simulink model "simulink_FCS_SDA"  (R2023a)
settings: Solver=VariableStepAuto  StartTime=0.0  StopTime=3*(1/freqHzSin)  FixedStep=Ts  RelTol=1e-3
InitFcn:
  | v0_setupFCS
StopFcn:
  | % t = table(out.seq, out.t_sim, 'VariableNames', ["Sequência de Vetores","Tempo de Simulação"]);
  | % writetable(t,'C:\Users\jpbru\OneDrive\Documentos\UFSC\COBEP 2023\sequencia_states.xlsx','Sheet','sim_CF_gw')
  | % winopen('C:\Users\jpbru\OneDrive\Documentos\UFSC\COBEP 2023\sequencia_states.xlsx')
  | %
  | % nome_arq = sprintf("gdq_caso-1_7.csv");
  | % writematrix([out.y_d out.y_q out.y_a out.y_b out.y_c out.ref_a out.ref_b out.ref_c],"C:\Users\jpbru\OneDrive\Documentos\MATLAB\CPBM\TrabFinal\Etapa 9 - Setembro2023 -\graficos\"+nome_arq)
  | 
  | sprintf("MSE = %.3f", out.mse)
  | sprintf("THD = %.3f", out.thd)
  | sprintf("Niter_avg = %d", round(out.Niter_avg))
  | % sprintf("Csw = %.0f", out.csw)
  | % sprintf("Tempo de Computo = %.3fms", out.tavg*1000)
values from neighbouring files (symbols this model uses):
  A = [A1; A2]    [v0_setupFCS.m]
  B = [B1; B2; B3; B4; B5; B6]    [v0_setupFCS.m]
  Csim = C*(1-P/100)    (= 5e-05)    [v0_setupFCS.m]
  dimA = length(A1)    [v0_setupFCS.m]
  dimB = length(B1)    [v0_setupFCS.m]
  freqHzSin = 50    [v0_setupFCS.m]
  Lsim = L*(1-P/100)    (= 0.002)    [v0_setupFCS.m]
  N = 4    [v0_setupFCS.m]
  N1 = 2    [v0_setupFCS.m]
  N2 = N+N1-1    (= 5)    [v0_setupFCS.m]
  Rsim = R*(1-P/100)    (= 60)    [v0_setupFCS.m]
  Ts = 1/Fs    (= 5e-05)    [v0_setupFCS.m]
  Vdc_sim = Vdc*1    (= 400)    [v0_setupFCS.m]
  vectors = [ 0   0   0 ... (first row only)    [v0_setupFCS.m]
  Vnoise = 0    [v0_setupFCS.m]
  Vo_ref_amp = 120*sqrt(2)    [v0_setupFCS.m]
undefined symbols (not defined in the file or in its folder): DiscIntNeverNeededParam, Lfilter
libraries: dspstat3 x10, spsSeriesRLCBranchLib x9, spsVoltageMeasurementLib x7, spsCurrentMeasurementLib x6, spsIdealSwitchLib x6, spsTHDLib x4, spsabctoAlphaBetaZeroLib x4, simulink x2, spsControlledVoltageSourceLib x1, sps_lib x1
settings Model: Creator=jpbru  LastModifiedBy=jpbru
settings SolverCC: AlgebraicLoopSolver=TrustRegion
settings DebuggingCC: UnconnectedInputMsg=warning  UnconnectedOutputMsg=warning  UnconnectedLineMsg=warning
settings ModelReferenceCC: EnableRefExpFcnMdlSchedulingChecks=on

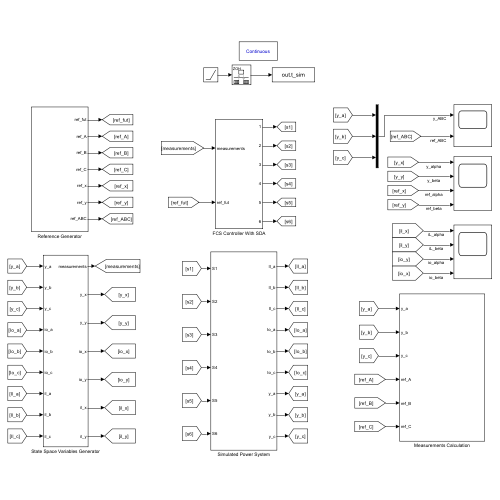
[thumbnail: Simulink's stored preview of the top-level diagram]
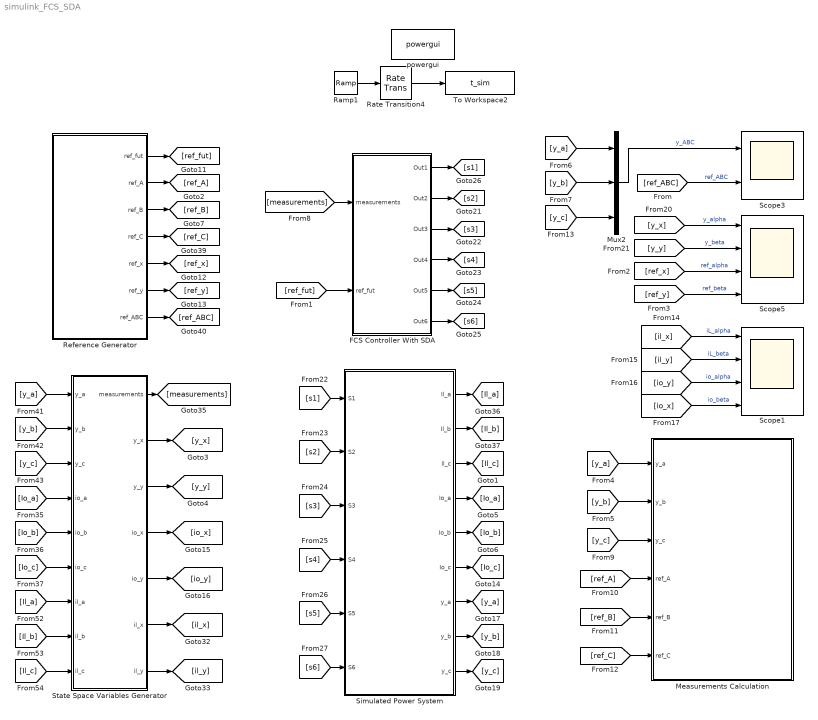
== system simulink_FCS_SDA ==
  FCS Controller With SDA : Subsystem
  Measurements Calculation : Subsystem
  Mux2 : Mux  Inputs=3
  Ramp1 : simulink/Sources/Ramp  slope=1  start=0  InitialOutput=0
  Rate Transition4 : RateTransition  OutPortSampleTime=Ts
  Reference Generator : Subsystem
  Scope1 : Scope  NumInputPorts=4
  Scope3 : Scope  NumInputPorts=2
  Scope5 : Scope  NumInputPorts=4
  Simulated Power System : Subsystem
  State Space Variables Generator : Subsystem
  To Workspace2 : ToWorkspace  VariableName=t_sim  SampleTime=Ts
      settings: Save2DSignal=2-D array (concatenate along first dimension)
  powergui : sps_lib/powergui  Priority=1  SimulationMode=Continuous  SampleTime=Ts  frequency=60  Iterations=50  frequencyindice=0  Pbase=100e6  ErrMax=1e-4  UnitsV=kV  UnitsW=MW  buscounter=0  FunctionMessages=off  echomessages=off  EnableUseOfTLC=off  CurrentSourceSwitches=off  DisableSnubberDevices=off  DisableRonSwitches=off  DisableVfSwitches=off  DisplayEquations=off  AutomaticDiscreteSolvers=off  SolverType=Tustin/Backward Euler (TBE)  Interpol=off  ExternalGateDelay=off  methode=off  Ts=100  x0status=blocks  SPID=on  SwTol=0  HookPort=off  NonlinearTolerance=1e-4  nMaxIteration=100  ContinueOnMaxIteration=off  RestoreLinks=warning  ResistiveCurrentMeasurement=off  Frange=[0:2:500]  Ylog=off  Xlog=on  ShowGrid=off  save=off  variable=ZData  structure=0  ZoomFFT=off  StartTime=0.0  cycles=1  DisplayStyle=1  fundamental=60  FreqAxis=off  MaxFrequency=1000  frequencyindicesteady=1  RmsSteady=1  display=off
  wires:
  [ref_y] -> Scope5/4  "ref_beta"
  [y_a] -> Mux2/1
  [y_b] -> Mux2/2
  [y_c] -> Mux2/3
  Mux2/1 -> Scope3/1  "y_ABC"
  [y_x] -> Scope5/1  "y_alpha"
  [y_y] -> Scope5/2  "y_beta"
  [ref_x] -> Scope5/3  "ref_alpha"
  Ramp1/1 -> Rate Transition4/1
  Rate Transition4/1 -> To Workspace2/1
  Reference Generator/1(ref_fut) -> [ref_fut]
  Reference Generator/2(ref_A) -> [ref_A]
  Reference Generator/3(ref_B) -> [ref_B]
  Reference Generator/4(ref_C) -> [ref_C]
  Reference Generator/6(ref_y) -> [ref_y]
  Reference Generator/5(ref_x) -> [ref_x]
  [y_a] -> State Space Variables Generator/1(y_a)
  [y_b] -> State Space Variables Generator/2(y_b)
  [y_c] -> State Space Variables Generator/3(y_c)
  [Io_a] -> State Space Variables Generator/4(io_a)
  [Io_b] -> State Space Variables Generator/5(io_b)
  [Io_c] -> State Space Variables Generator/6(io_c)
  [Il_a] -> State Space Variables Generator/7(il_a)
  [Il_b] -> State Space Variables Generator/8(il_b)
  [Il_c] -> State Space Variables Generator/9(il_c)
  State Space Variables Generator/1(measurements) -> [measurements]
  State Space Variables Generator/4(io_x) -> [io_x]
  State Space Variables Generator/5(io_y) -> [io_y]
  State Space Variables Generator/6(il_x) -> [il_x]
  State Space Variables Generator/7(il_y) -> [il_y]
  State Space Variables Generator/3(y_y) -> [y_y]
  State Space Variables Generator/2(y_x) -> [y_x]
  Reference Generator/7(ref_ABC) -> [ref_ABC]
  [ref_ABC] -> Scope3/2  "ref_ABC"
  [measurements] -> FCS Controller With SDA/1(measurements)
  [ref_fut] -> FCS Controller With SDA/2(ref_fut)
  FCS Controller With SDA/1(Out1) -> [s1]
  FCS Controller With SDA/2(Out2) -> [s2]
  FCS Controller With SDA/3(Out3) -> [s3]
  FCS Controller With SDA/4(Out4) -> [s4]
  FCS Controller With SDA/5(Out5) -> [s5]
  FCS Controller With SDA/6(Out6) -> [s6]
  [s1] -> Simulated Power System/1(S1)
  Simulated Power System/9(y_c) -> [y_c]
  Simulated Power System/8(y_b) -> [y_b]
  Simulated Power System/7(y_a) -> [y_a]
  [s2] -> Simulated Power System/2(S2)
  [s3] -> Simulated Power System/3(S3)
  [s4] -> Simulated Power System/4(S4)
  [s5] -> Simulated Power System/5(S5)
  [s6] -> Simulated Power System/6(S6)
  Simulated Power System/1(Il_a) -> [Il_a]
  Simulated Power System/2(Il_b) -> [Il_b]
  Simulated Power System/3(Il_c) -> [Il_c]
  Simulated Power System/4(Io_a) -> [Io_a]
  Simulated Power System/5(Io_b) -> [Io_b]
  Simulated Power System/6(Io_c) -> [Io_c]
  [ref_C] -> Measurements Calculation/6(ref_C)
  [ref_B] -> Measurements Calculation/5(ref_B)
  [ref_A] -> Measurements Calculation/4(ref_A)
  [y_c] -> Measurements Calculation/3(y_c)
  [y_b] -> Measurements Calculation/2(y_b)
  [y_a] -> Measurements Calculation/1(y_a)
  [il_x] -> Scope1/1  "iL_alpha"
  [il_y] -> Scope1/2  "iL_beta"
  [io_y] -> Scope1/3  "io_alpha"
  [io_x] -> Scope1/4  "io_beta"

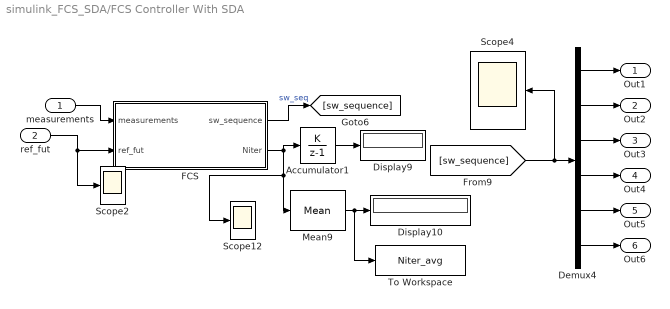
== system simulink_FCS_SDA/FCS Controller With SDA ==
  measurements : Inport
  ref_fut : Inport  Port=2
  Accumulator1 : DiscreteIntegrator  IntegratorMethod=Accumulation: Forward Euler  SampleTime=Ts  ICPrevOutput=DiscIntNeverNeededParam  ICPrevScaledInput=DiscIntNeverNeededParam
  Demux4 : Demux  Outputs=6
  Display10 : Display
  Display9 : Display
  FCS : MATLAB Function  TreatAsAtomicUnit=on  SystemSampleTime=Ts
  Mean9 : dspstat3/Mean  run=on  reset_popup=None  directionMode=Each column  dimension=1  roiEnable=off  roiType=Rectangles  roiPortion=Entire ROI  roiOutput=Individual statistics for each ROI  roiFlag=off  roundingMode=Floor  overflowMode=off  outputDataTypeStr=Inherit: Same as accumulator  outputMin=[]  outputMax=[]  outputLastDataTypeStr=Inherit: Same as accumulator
  Scope12 : Scope
  Scope2 : Scope
  Scope4 : Scope
  To Workspace : ToWorkspace  VariableName=Niter_avg  SampleTime=-1
      settings: MaxDataPoints=1
  Out1 : Outport
  Out2 : Outport  Port=2
  Out3 : Outport  Port=3
  Out4 : Outport  Port=4
  Out5 : Outport  Port=5
  Out6 : Outport  Port=6
  wires:
  Demux4/5 -> Out5/1
  [sw_sequence] -> Scope4/1, Demux4/1
  FCS/1(sw_sequence) -> [sw_sequence]  "sw_seq"
  Demux4/1 -> Out1/1
  FCS/2(Niter) -> Accumulator1/1, Scope12/1, Mean9/1
  ref_fut/1 -> Scope2/1, FCS/2(ref_fut)
  Mean9/1 -> To Workspace/1, Display10/1
  Accumulator1/1 -> Display9/1
  measurements/1 -> FCS/1(measurements)
  Demux4/3 -> Out3/1
  Demux4/2 -> Out2/1
  Demux4/6 -> Out6/1
  Demux4/4 -> Out4/1

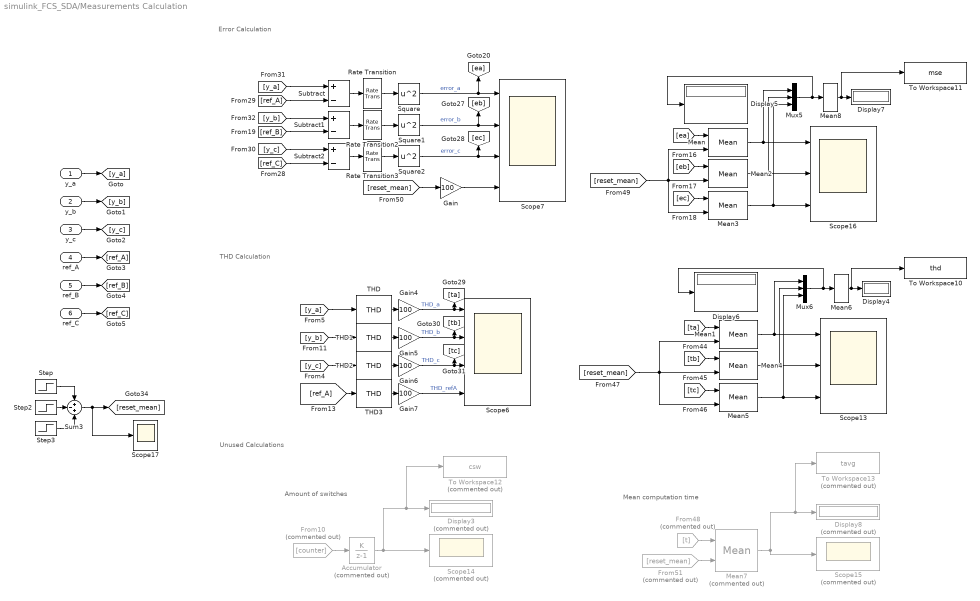
== system simulink_FCS_SDA/Measurements Calculation ==
  note: Unused Calculations
  note: THD Calculation
  note: Error Calculation
  note: Mean computation time
  note: Amount of switches
  y_a : Inport
  y_b : Inport  Port=2
  y_c : Inport  Port=3
  ref_A : Inport  Port=4
  ref_B : Inport  Port=5
  ref_C : Inport  Port=6
  Accumulator : DiscreteIntegrator  Commented=on  IntegratorMethod=Accumulation: Forward Euler  SampleTime=-1  ICPrevOutput=DiscIntNeverNeededParam  ICPrevScaledInput=DiscIntNeverNeededParam
  Display3 : Display  Commented=on
  Display{4..7} (4 alike) : Display
  Display8 : Display  Commented=on
      settings: Format=short_e
  From10 : From  Commented=on  GotoTag=counter
  From48 : From  Commented=on  GotoTag=t
  From51 : From  Commented=on  GotoTag=reset_mean
  Gain{,4..7} (5 alike) : Gain  Gain=100
  Mean{,1..5} (6 alike) : dspstat3/Mean  run=on  reset_popup=Rising edge  directionMode=Each column  dimension=1  roiEnable=off  roiType=Rectangles  roiPortion=Entire ROI  roiOutput=Individual statistics for each ROI  roiFlag=off  roundingMode=Floor  overflowMode=off  outputDataTypeStr=Inherit: Same as accumulator  outputMin=[]  outputMax=[]  outputLastDataTypeStr=Inherit: Same as accumulator
  Mean6 : dspstat3/Mean  run=off  reset_popup=Rising edge  directionMode=Entire input  dimension=1  roiEnable=off  roiType=Rectangles  roiPortion=Entire ROI  roiOutput=Individual statistics for each ROI  roiFlag=off  roundingMode=Floor  overflowMode=off  outputDataTypeStr=Inherit: Same as accumulator  outputMin=[]  outputMax=[]  outputLastDataTypeStr=Inherit: Same as accumulator
  Mean7 : dspstat3/Mean  Commented=on  run=on  reset_popup=Rising edge  directionMode=Each column  dimension=1  roiEnable=off  roiType=Rectangles  roiPortion=Entire ROI  roiOutput=Individual statistics for each ROI  roiFlag=off  roundingMode=Floor  overflowMode=off  outputDataTypeStr=Inherit: Same as accumulator  outputMin=[]  outputMax=[]  outputLastDataTypeStr=Inherit: Same as accumulator
  Mean8 : dspstat3/Mean  run=off  reset_popup=Rising edge  directionMode=Entire input  dimension=1  roiEnable=off  roiType=Rectangles  roiPortion=Entire ROI  roiOutput=Individual statistics for each ROI  roiFlag=off  roundingMode=Floor  overflowMode=off  outputDataTypeStr=Inherit: Same as accumulator  outputMin=[]  outputMax=[]  outputLastDataTypeStr=Inherit: Same as accumulator
  Mux5 : Mux  Inputs=3
  Mux6 : Mux  Inputs=3
  Rate Transition : RateTransition  OutPortSampleTime=Ts
  Rate Transition2 : RateTransition  OutPortSampleTime=Ts
  Rate Transition3 : RateTransition  OutPortSampleTime=Ts
  Scope13 : Scope  NumInputPorts=3
  Scope14 : Scope  Commented=on
  Scope15 : Scope  Commented=on
  Scope16 : Scope  NumInputPorts=3
  Scope17 : Scope
  Scope6 : Scope  NumInputPorts=4
  Scope7 : Scope  NumInputPorts=4
  Square : Math  Operator=square
  Square1 : Math  Operator=square
  Square2 : Math  Operator=square
  Step : Step  Time=(1/freqHzSin)  SampleTime=Ts
  Step2 : Step  Time=(1/freqHzSin)+Ts  SampleTime=Ts
  Step3 : Step  Time=(1/freqHzSin)*2  SampleTime=Ts
  Subtract : Sum  Inputs=+-
  Subtract1 : Sum  Inputs=+-
  Subtract2 : Sum  Inputs=+-
  Sum3 : Sum  Inputs=+-+
  THD{,1..3} (4 alike) : spsTHDLib/THD  Freq=50  Ts=Ts
  To Workspace10 : ToWorkspace  VariableName=thd  SampleTime=-1
      settings: MaxDataPoints=1
  To Workspace11 : ToWorkspace  VariableName=mse  SampleTime=-1
      settings: MaxDataPoints=1
  To Workspace12 : ToWorkspace  Commented=on  VariableName=csw  SampleTime=-1
      settings: MaxDataPoints=1
  To Workspace13 : ToWorkspace  Commented=on  VariableName=tavg  SampleTime=-1
      settings: MaxDataPoints=1
  wires:
  Rate Transition2/1 -> Square1/1
  Gain5/1 -> [tb], Scope6/2  "THD_b"
  Mean8/1 -> To Workspace11/1, Display7/1
  Mean7/1 -> To Workspace13/1, Display8/1, Scope15/1
  Subtract2/1 -> Rate Transition3/1
  Sum3/1 -> Scope17/1, [reset_mean]
  Mean6/1 -> To Workspace10/1, Display4/1
  Gain6/1 -> [tc], Scope6/3  "THD_c"
  THD2/1 -> Gain6/1
  Mux5/1 -> Mean8/1, Display5/1
  Mean3/1 -> Mux5/3, Scope16/3
  Accumulator/1 -> To Workspace12/1, Display3/1, Scope14/1
  [tc] -> Mean5/1
  [eb] -> Mean2/1
  Mux6/1 -> Display6/1, Mean6/1
  Mean5/1 -> Mux6/3, Scope13/3
  Square2/1 -> [ec], Scope7/3  "error_c"
  [ta] -> Mean1/1
  Gain4/1 -> [ta], Scope6/1  "THD_a"
  Mean1/1 -> Mux6/1, Scope13/1
  [ref_A] -> THD3/1
  [ref_C] -> Subtract2/2
  From48/1 -> Mean7/1
  Square/1 -> [ea], Scope7/1  "error_a"
  Rate Transition3/1 -> Square2/1
  [y_a] -> THD/1
  Subtract/1 -> Rate Transition/1
  [tb] -> Mean4/1
  From10/1 -> Accumulator/1
  [y_b] -> Subtract1/1
  [reset_mean] -> Mean3/2, Mean2/2, Mean/2
  Step2/1 -> Sum3/2
  Step3/1 -> Sum3/3
  [reset_mean] -> Mean1/2, Mean5/2, Mean4/2
  [reset_mean] -> Gain/1
  Mean2/1 -> Mux5/2, Scope16/2
  Mean/1 -> Mux5/1, Scope16/1
  [ec] -> Mean3/1
  [ea] -> Mean/1
  [y_b] -> THD1/1
  Gain7/1 -> Scope6/4  "THD_refA"
  [y_c] -> Subtract2/1
  Square1/1 -> [eb], Scope7/2  "error_b"
  [ref_A] -> Subtract/2
  [ref_B] -> Subtract1/2
  Subtract1/1 -> Rate Transition2/1
  THD/1 -> Gain4/1
  THD1/1 -> Gain5/1
  THD3/1 -> Gain7/1
  [y_c] -> THD2/1
  Gain/1 -> Scope7/4
  Rate Transition/1 -> Square/1
  [y_a] -> Subtract/1
  Step/1 -> Sum3/1
  From51/1 -> Mean7/2
  Mean4/1 -> Mux6/2, Scope13/2
  ref_C/1 -> [ref_C]
  ref_B/1 -> [ref_B]
  ref_A/1 -> [ref_A]
  y_c/1 -> [y_c]
  y_b/1 -> [y_b]
  y_a/1 -> [y_a]

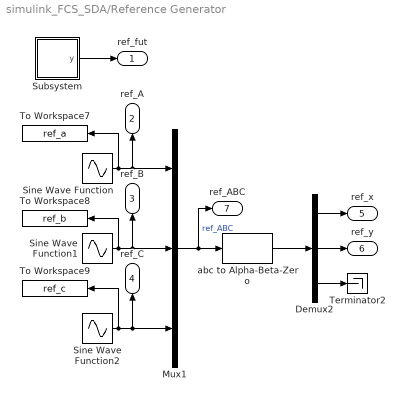
== system simulink_FCS_SDA/Reference Generator ==
  Demux2 : Demux  Outputs=3
  Mux1 : Mux  Inputs=3
  Sine Wave Function : Sin  Amplitude=Vo_ref_amp  Frequency=2*pi*50  SampleTime=Ts
  Sine Wave Function1 : Sin  Amplitude=Vo_ref_amp  Frequency=2*pi*50  Phase=-2*pi/3  SampleTime=Ts
  Sine Wave Function2 : Sin  Amplitude=Vo_ref_amp  Frequency=2*pi*50  Phase=2*pi/3  SampleTime=Ts
  Subsystem : Subsystem
  Terminator2 : Terminator
  To Workspace7 : ToWorkspace  VariableName=ref_a  SampleTime=Ts
      settings: Save2DSignal=2-D array (concatenate along first dimension)
  To Workspace8 : ToWorkspace  VariableName=ref_b  SampleTime=Ts
      settings: Save2DSignal=2-D array (concatenate along first dimension)
  To Workspace9 : ToWorkspace  VariableName=ref_c  SampleTime=Ts
      settings: Save2DSignal=2-D array (concatenate along first dimension)
  abc to Alpha-Beta-Zero : spsabctoAlphaBetaZeroLib/abc to Alpha-Beta-Zero
  ref_fut : Outport
  ref_A : Outport  Port=2
  ref_B : Outport  Port=3
  ref_C : Outport  Port=4
  ref_x : Outport  Port=5
  ref_y : Outport  Port=6
  ref_ABC : Outport  Port=7
  wires:
  Subsystem/1(y) -> ref_fut/1
  Demux2/2 -> ref_y/1
  Sine Wave Function/1 -> Mux1/1, ref_A/1, To Workspace7/1
  Demux2/3 -> Terminator2/1
  Sine Wave Function1/1 -> Mux1/2, ref_B/1, To Workspace8/1
  Demux2/1 -> ref_x/1
  Sine Wave Function2/1 -> Mux1/3, ref_C/1, To Workspace9/1
  Mux1/1 -> ref_ABC/1, abc to Alpha-Beta-Zero/1  "ref_ABC"
  abc to Alpha-Beta-Zero/1 -> Demux2/1

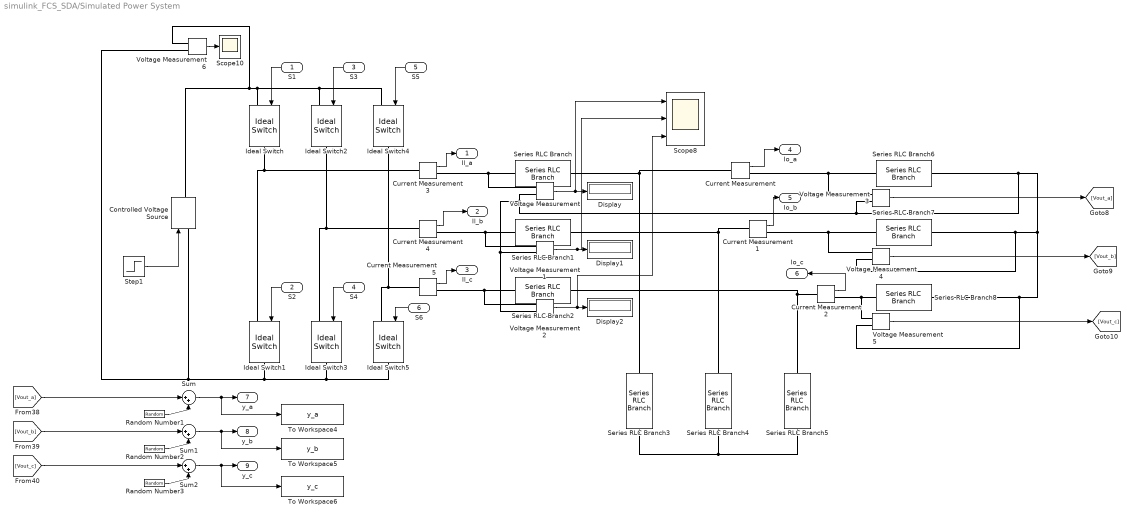
== system simulink_FCS_SDA/Simulated Power System ==
  S1 : Inport
  S2 : Inport  Port=2
  S3 : Inport  Port=3
  S4 : Inport  Port=4
  S5 : Inport  Port=5
  S6 : Inport  Port=6
  Controlled Voltage Source : spsControlledVoltageSourceLib/Controlled Voltage Source  Initialize=on  Source_Type=DC  Amplitude=Vdc_sim  Phase=0  Frequency=0  Measurements=None
  Current Measurement{,1..5} (6 alike) : spsCurrentMeasurementLib/Current Measurement  PhasorSimulation=off  OutputType=Complex  PSBequivalent=0
  Display : Display
  Display1 : Display
  Display2 : Display
  Ideal Switch{,1..5} (6 alike) : spsIdealSwitchLib/Ideal Switch  Ron=0.001  Lon=0  IC=0  Rs=1e5  Cs=inf  Measurements=off
  Random Number1 : RandomNumber  Variance=Vnoise  SampleTime=Ts
  Random Number2 : RandomNumber  Variance=Vnoise  SampleTime=Ts
  Random Number3 : RandomNumber  Variance=Vnoise  SampleTime=Ts
  Scope10 : Scope
  Scope8 : Scope  NumInputPorts=3
  Series RLC Branch : spsSeriesRLCBranchLib/Series RLC Branch  LConnTagsString=__new0  RConnTagsString=__new0  BranchType=L  Resistance=1  Inductance=Lsim  SetiL0=off  InitialCurrent=0  Capacitance=1e-6  Setx0=off  InitialVoltage=0  Measurements=None
  Series RLC Branch1 : spsSeriesRLCBranchLib/Series RLC Branch  LConnTagsString=__new0  RConnTagsString=__new0  BranchType=L  Resistance=1  Inductance=Lsim  SetiL0=off  InitialCurrent=0  Capacitance=1e-6  Setx0=off  InitialVoltage=0  Measurements=None
  Series RLC Branch2 : spsSeriesRLCBranchLib/Series RLC Branch  LConnTagsString=__new0  RConnTagsString=__new0  BranchType=L  Resistance=1  Inductance=Lsim  SetiL0=off  InitialCurrent=0  Capacitance=1e-6  Setx0=off  InitialVoltage=0  Measurements=None
  Series RLC Branch3 : spsSeriesRLCBranchLib/Series RLC Branch  LConnTagsString=__new0  RConnTagsString=__new0  BranchType=C  Resistance=1  Inductance=1e-3  SetiL0=off  InitialCurrent=0  Capacitance=Csim  Setx0=off  InitialVoltage=0  Measurements=None
  Series RLC Branch4 : spsSeriesRLCBranchLib/Series RLC Branch  LConnTagsString=__new0  RConnTagsString=__new0  BranchType=C  Resistance=1  Inductance=1e-3  SetiL0=off  InitialCurrent=0  Capacitance=Csim  Setx0=off  InitialVoltage=0  Measurements=None
  Series RLC Branch5 : spsSeriesRLCBranchLib/Series RLC Branch  LConnTagsString=__new0  RConnTagsString=__new0  BranchType=C  Resistance=1  Inductance=1e-3  SetiL0=off  InitialCurrent=0  Capacitance=Csim  Setx0=off  InitialVoltage=0  Measurements=None
  Series RLC Branch6 : spsSeriesRLCBranchLib/Series RLC Branch  LConnTagsString=__new0  RConnTagsString=__new0  BranchType=R  Resistance=Rsim  Inductance=Lfilter  SetiL0=off  InitialCurrent=0  Capacitance=1e-6  Setx0=off  InitialVoltage=0  Measurements=None
  Series RLC Branch7 : spsSeriesRLCBranchLib/Series RLC Branch  LConnTagsString=__new0  RConnTagsString=__new0  BranchType=R  Resistance=Rsim  Inductance=Lfilter  SetiL0=off  InitialCurrent=0  Capacitance=1e-6  Setx0=off  InitialVoltage=0  Measurements=None
  Series RLC Branch8 : spsSeriesRLCBranchLib/Series RLC Branch  LConnTagsString=__new0  RConnTagsString=__new0  BranchType=R  Resistance=Rsim  Inductance=Lfilter  SetiL0=off  InitialCurrent=0  Capacitance=1e-6  Setx0=off  InitialVoltage=0  Measurements=None
  Step1 : Step  Time=0.5  Before=Vdc_sim  After=Vdc_sim  SampleTime=Ts
  Sum : Sum  Inputs=|++
  Sum1 : Sum  Inputs=|++
  Sum2 : Sum  Inputs=|++
  To Workspace4 : ToWorkspace  VariableName=y_a  SampleTime=Ts
      settings: Save2DSignal=2-D array (concatenate along first dimension)
  To Workspace5 : ToWorkspace  VariableName=y_b  SampleTime=Ts
      settings: Save2DSignal=2-D array (concatenate along first dimension)
  To Workspace6 : ToWorkspace  VariableName=y_c  SampleTime=Ts
      settings: Save2DSignal=2-D array (concatenate along first dimension)
  Voltage Measurement{,1..6} (7 alike) : spsVoltageMeasurementLib/Voltage Measurement  PhasorSimulation=off  OutputType=Complex  PSBequivalent=0
  Il_a : Outport
  Il_b : Outport  Port=2
  Il_c : Outport  Port=3
  Io_a : Outport  Port=4
  Io_b : Outport  Port=5
  Io_c : Outport  Port=6
  y_a : Outport  Port=7
  y_b : Outport  Port=8
  y_c : Outport  Port=9
  wires:
  Step1/1 -> Controlled Voltage Source/1
  Sum1/1 -> y_b/1, To Workspace5/1
  Random Number3/1 -> Sum2/2
  Sum2/1 -> y_c/1, To Workspace6/1
  Random Number2/1 -> Sum1/2
  Voltage Measurement/1 -> Scope8/1, Display/1
  Sum/1 -> y_a/1, To Workspace4/1
  Voltage Measurement2/1 -> Scope8/3, Display2/1
  Current Measurement1/1 -> Io_b/1
  [Vout_c] -> Sum2/1
  Voltage Measurement1/1 -> Scope8/2, Display1/1
  Voltage Measurement6/1 -> Scope10/1
  Random Number1/1 -> Sum/2
  [Vout_b] -> Sum1/1
  Current Measurement2/1 -> Io_c/1
  Current Measurement4/1 -> Il_b/1
  Current Measurement3/1 -> Il_a/1
  [Vout_a] -> Sum/1
  Current Measurement5/1 -> Il_c/1
  Current Measurement/1 -> Io_a/1
  S1/1 -> Ideal Switch/1
  S3/1 -> Ideal Switch2/1
  S5/1 -> Ideal Switch4/1
  S2/1 -> Ideal Switch1/1
  S4/1 -> Ideal Switch3/1
  S6/1 -> Ideal Switch5/1
  Voltage Measurement3/1 -> [Vout_a]
  Voltage Measurement4/1 -> [Vout_b]
  Voltage Measurement5/1 -> [Vout_c]
  connections:
  Voltage Measurement3/LConn1 -- Current Measurement/RConn1 -- Series RLC Branch6/LConn1
  Ideal Switch/LConn1 -- Ideal Switch4/LConn1 -- Ideal Switch2/LConn1 -- Controlled Voltage Source/RConn1 -- Voltage Measurement6/LConn1
  Series RLC Branch6/RConn1 -- Voltage Measurement2/LConn2 -- Voltage Measurement1/LConn2 -- Voltage Measurement/LConn2 -- Voltage Measurement3/LConn2 -- Voltage Measurement4/LConn2 -- Series RLC Branch7/RConn1 -- Voltage Measurement5/LConn2 -- Series RLC Branch8/RConn1
  Series RLC Branch5/LConn1 -- Current Measurement2/LConn1 -- Series RLC Branch2/RConn1
  Ideal Switch1/RConn1 -- Controlled Voltage Source/LConn1 -- Voltage Measurement6/LConn2 -- Ideal Switch5/RConn1 -- Ideal Switch3/RConn1
  Series RLC Branch2/LConn1 -- Current Measurement5/RConn1 -- Voltage Measurement2/LConn1
  Series RLC Branch/RConn1 -- Current Measurement/LConn1 -- Series RLC Branch3/LConn1
  Ideal Switch/RConn1 -- Current Measurement3/LConn1 -- Ideal Switch1/LConn1
  Series RLC Branch/LConn1 -- Current Measurement3/RConn1 -- Voltage Measurement/LConn1
  Ideal Switch3/LConn1 -- Current Measurement4/LConn1 -- Ideal Switch2/RConn1
  Series RLC Branch4/LConn1 -- Current Measurement1/LConn1 -- Series RLC Branch1/RConn1
  Series RLC Branch7/LConn1 -- Current Measurement1/RConn1 -- Voltage Measurement4/LConn1
  Series RLC Branch8/LConn1 -- Current Measurement2/RConn1 -- Voltage Measurement5/LConn1
  Series RLC Branch3/RConn1 -- Series RLC Branch5/RConn1 -- Series RLC Branch4/RConn1
  Ideal Switch5/LConn1 -- Current Measurement5/LConn1 -- Ideal Switch4/RConn1
  Series RLC Branch1/LConn1 -- Current Measurement4/RConn1 -- Voltage Measurement1/LConn1

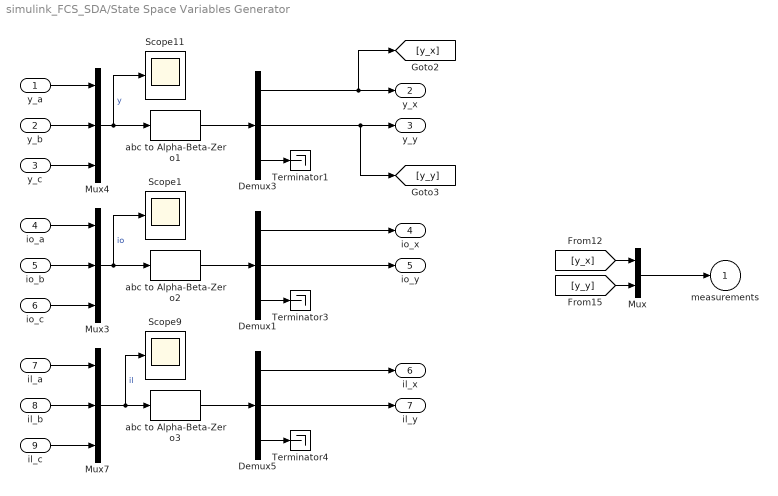
== system simulink_FCS_SDA/State Space Variables Generator ==
  y_a : Inport
  y_b : Inport  Port=2
  y_c : Inport  Port=3
  io_a : Inport  Port=4
  io_b : Inport  Port=5
  io_c : Inport  Port=6
  il_a : Inport  Port=7
  il_b : Inport  Port=8
  il_c : Inport  Port=9
  Demux1 : Demux  Outputs=3
  Demux3 : Demux  Outputs=3
  Demux5 : Demux  Outputs=3
  Mux : Mux  Inputs=2
  Mux3 : Mux  Inputs=3
  Mux4 : Mux  Inputs=3
  Mux7 : Mux  Inputs=3
  Scope1 : Scope
  Scope11 : Scope
  Scope9 : Scope
  Terminator1 : Terminator
  Terminator3 : Terminator
  Terminator4 : Terminator
  abc to Alpha-Beta-Zero1 : spsabctoAlphaBetaZeroLib/abc to Alpha-Beta-Zero
  abc to Alpha-Beta-Zero2 : spsabctoAlphaBetaZeroLib/abc to Alpha-Beta-Zero
  abc to Alpha-Beta-Zero3 : spsabctoAlphaBetaZeroLib/abc to Alpha-Beta-Zero
  measurements : Outport
  y_x : Outport  Port=2
  y_y : Outport  Port=3
  io_x : Outport  Port=4
  io_y : Outport  Port=5
  il_x : Outport  Port=6
  il_y : Outport  Port=7
  wires:
  Demux3/1 -> [y_x], y_x/1
  Demux3/3 -> Terminator1/1
  Mux7/1 -> Scope9/1, abc to Alpha-Beta-Zero3/1  "il"
  Mux4/1 -> Scope11/1, abc to Alpha-Beta-Zero1/1  "y"
  il_c/1 -> Mux7/3
  Demux3/2 -> [y_y], y_y/1
  abc to Alpha-Beta-Zero1/1 -> Demux3/1
  io_a/1 -> Mux3/1
  abc to Alpha-Beta-Zero2/1 -> Demux1/1
  [y_x] -> Mux/1
  Mux3/1 -> Scope1/1, abc to Alpha-Beta-Zero2/1  "io"
  io_b/1 -> Mux3/2
  y_c/1 -> Mux4/3
  Demux1/2 -> io_y/1
  Demux1/1 -> io_x/1
  abc to Alpha-Beta-Zero3/1 -> Demux5/1
  Demux5/2 -> il_y/1
  Demux5/1 -> il_x/1
  Demux5/3 -> Terminator4/1
  io_c/1 -> Mux3/3
  Demux1/3 -> Terminator3/1
  y_a/1 -> Mux4/1
  il_b/1 -> Mux7/2
  il_a/1 -> Mux7/1
  y_b/1 -> Mux4/2
  Mux/1 -> measurements/1
  [y_y] -> Mux/2

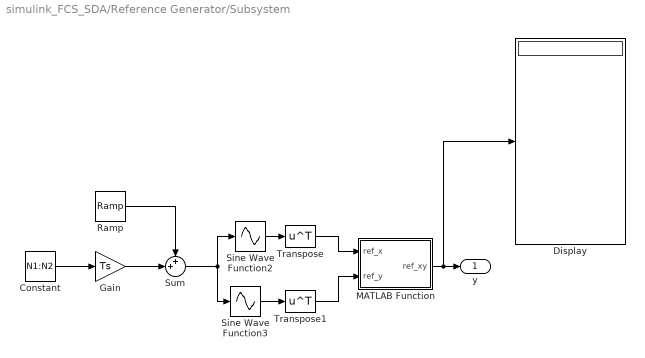
== system simulink_FCS_SDA/Reference Generator/Subsystem ==
  Constant : Constant  Value=N1:N2
  Display : Display
  Gain : Gain  Gain=Ts
  MATLAB Function : MATLAB Function  TreatAsAtomicUnit=on
  Ramp : simulink/Sources/Ramp  slope=1  start=0  InitialOutput=0
  Sine Wave Function2 : Sin  TimeSource=Use external signal  Amplitude=Vo_ref_amp  Frequency=2*pi*50  SampleTime=Ts
  Sine Wave Function3 : Sin  TimeSource=Use external signal  Amplitude=Vo_ref_amp  Frequency=2*pi*50  Phase=-pi/2  SampleTime=Ts
  Sum : Sum  Inputs=++|
  Transpose : Math  Operator=transpose
  Transpose1 : Math  Operator=transpose
  y : Outport
  wires:
  Sine Wave Function2/1 -> Transpose/1
  Sum/1 -> Sine Wave Function3/1, Sine Wave Function2/1
  Ramp/1 -> Sum/1
  Gain/1 -> Sum/2
  Constant/1 -> Gain/1
  Sine Wave Function3/1 -> Transpose1/1
  Transpose/1 -> MATLAB Function/1(ref_x)
  Transpose1/1 -> MATLAB Function/2(ref_y)
  MATLAB Function/1(ref_xy) -> Display/1, y/1

== matlab function simulink_FCS_SDA/FCS Controller With SDA/FCS ==
  settings: updateMethod=DISCRETE  sampleTime=Ts
  data: measurements input; sw_sequence output; ref_fut input; Niter output; A parameter; B parameter; dimA parameter; dimB parameter; vectors parameter; N1 parameter; N parameter
%function[variáveis que envia pra fora do bloco na simulação] = fcn(entradas(com conexões físicas) e parâmetros(que são pegos da workspace))
function [sw_sequence, Niter] = fcn(measurements, ref_fut, A, B, dimA, dimB, vectors, N1, N) 
% coder.extrinsic("combn");
persistent t  y_ant s_ant %variáveis que mantém o valor entre os loops
if isempty(t) %caso t ainda não tenha valor definido
    t = 0; %o primeiro loop assume t=0
    s_ant = zeros(3,dimB);
    y_ant = zeros(2,dimA-1);
else %caso não seja o primeiro loop
    t = t + 1; %t vai incrementando em cada loop
    y_ant(:,end:-1:2) = y_ant(:,end-1:-1:1);
end
y_ant(:,1) = measurements;
y_comp = zeros(2,size(y_ant,2)+N1-1+N); %size(y_ant,2) => old y's; (N1-1)=>if N1=2, 1 more cell to store in k+1; N => to store N predictions of output 
y_comp(:,N+N1:end) = y_ant;
y_ref = ref_fut;

Niter = 0;
J_opt = inf;
s = zeros(3,N);
index = ones(N,1);
s_opt = s_ant(:,1);
y_calc = zeros(2,1);
sw_sequence = zeros(6,1);%vetor que define o estado de cada uma das 6 chaves para aplicar nessa amostra

%% Apply the computed switching states
if N1 == 2
    for aux = 1:3 %loop para definir o vetor
        sw_sequence(2*aux-1) = s_ant(aux,1); 
        sw_sequence(2*aux) = not(s_ant(aux,1));
    end
    y_calc(1) = -A(1,2:end)*y_comp(1,N+N1:end)' + B(1,:)*s_ant(1,:)' + B(2,:)*s_ant(2,:)' + B(3,:)*s_ant(3,:)';
    y_calc(2) = -A(2,2:end)*y_comp(2,N+N1:end)' + B(4,:)*s_ant(1,:)' + B(5,:)*s_ant(2,:)' + B(6,:)*s_ant(3,:)';
    y_comp(:,N+1) = y_calc;
end

calc_vec = true;
while calc_vec
   J = 0;
   for horizon = 1:N
       Niter = Niter + 1;
       s_comp = [s(:,end-horizon+1:end) s_ant(:,1:dimB-horizon)];
       y_calc(1) = -A(1,2:end)*y_comp(1,N+1-(horizon-1):end-(N1-1)-(horizon-1))' + B(1,:)*s_comp(1,:)' + B(2,:)*s_comp(2,:)' + B(3,:)*s_comp(3,:)'; 
       y_calc(2) = -A(2,2:end)*y_comp(2,N+1-(horizon-1):end-(N1-1)-(horizon-1))' + B(4,:)*s_comp(1,:)' + B(5,:)*s_comp(2,:)' + B(6,:)*s_comp(3,:)';
       y_comp(:,N-(horizon-1)) = y_calc;
       
       J = J + (y_ref(1,horizon)-y_calc(1))^2+(y_ref(2,horizon)-y_calc(2))^2;
       if horizon == N
            J = sqrt(J);
       end
       if J < J_opt
           J_opt = J;
           s_opt = s(:,N);
       end
   end

   for aux = N:-1:1
        index(aux) = index(aux)+1;
        if index(aux) > size(vectors,1)
            if aux == 1
                calc_vec = false;
            else
                index(aux) = 1;
            end
        else
            for i = 1:N
                s(:,i) = vectors(index(i),:)';
            end
            break;
        end
   end
end

s_ant(:,end:-1:2) = s_ant(:,end-1:-1:1);
s_ant(:,1) = s_opt;

if N1 == 1
    for aux = 1:3 %loop para definir o vetor
        sw_sequence(2*aux-1) = s_ant(aux,1); 
        sw_sequence(2*aux) = not(s_ant(aux,1));
    end
end

== matlab function simulink_FCS_SDA/Reference Generator/Subsystem/MATLAB Function ==
  data: ref_x input; ref_y input; ref_xy output
function ref_xy = fcn(ref_x, ref_y)

ref_xy = [ref_x;ref_y];
